simulink model "BierPong_02"  (R2021a)
settings: Solver=VariableStepAuto  StartTime=0.0  StopTime=5.0  RelTol=1e-3
model workspace (MAT data in the model file):
  c_w = 0.47
  d_Ball = 0.04
  d_cup = 0.095
  g = 9.81
  len = 2.1
  m_Ball = 2.7
  roh = 1.2
  s_cup = 0.05
settings Model: OrderedModelArguments=off  Creator=Max  LastModifiedBy=Max

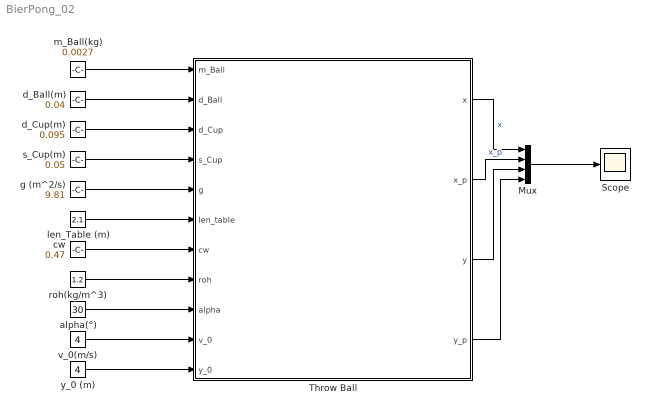
== system BierPong_02 ==
  Mux : Mux
  Scope : Scope
  Throw Ball : Subsystem
  alpha(°) : Constant  Value=30
  cw : Constant  Value=0.47
  d_Ball(m) : Constant  Value=0.04
  d_Cup(m) : Constant  Value=0.095
  g (m^2/s) : Constant  Value=9.81
  len_Table (m) : Constant  Value=2.1
  m_Ball(kg) : Constant  Value=0.0027
  roh(kg/m^3) : Constant  Value=1.2
  s_Cup(m) : Constant  Value=0.05
  v_0(m/s) : Constant  Value=4
  y_0 (m) : Constant  Value=4
  wires:
  m_Ball(kg)/1 -> Throw Ball/1(m_Ball)
  d_Ball(m)/1 -> Throw Ball/2(d_Ball)
  d_Cup(m)/1 -> Throw Ball/3(d_Cup)
  s_Cup(m)/1 -> Throw Ball/4(s_Cup)
  roh(kg/m^3)/1 -> Throw Ball/8(roh)
  cw/1 -> Throw Ball/7(cw)
  len_Table (m)/1 -> Throw Ball/6(len_table)
  g (m^2/s)/1 -> Throw Ball/5(g)
  Throw Ball/1(x) -> Mux/1  "x"
  Throw Ball/2(x_p) -> Mux/2  "x_p"
  Throw Ball/3(y) -> Mux/3
  Throw Ball/4(y_p) -> Mux/4
  Mux/1 -> Scope/1
  alpha(°)/1 -> Throw Ball/9(alpha)
  v_0(m/s)/1 -> Throw Ball/10(v_0)
  y_0 (m)/1 -> Throw Ball/11(y_0)

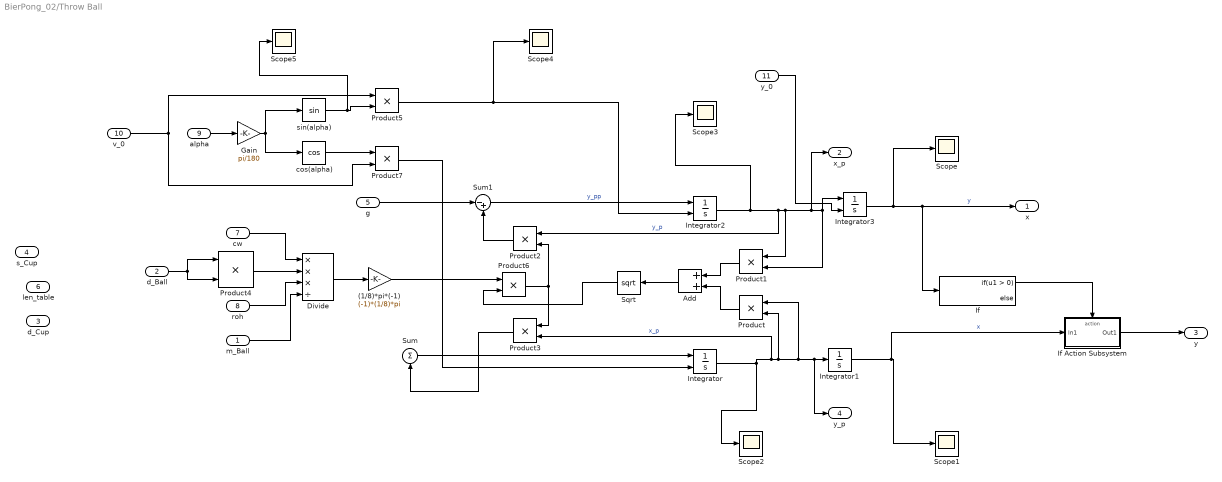
== system BierPong_02/Throw Ball ==
  m_Ball : Inport
  d_Ball : Inport  Port=2
  d_Cup : Inport  Port=3
  s_Cup : Inport  Port=4
  g : Inport  Port=5
  len_table : Inport  Port=6
  cw : Inport  Port=7
  roh : Inport  Port=8
  alpha : Inport  Port=9
  v_0 : Inport  Port=10
  y_0 : Inport  Port=11
  " sin(alpha)" : Trigonometry  OutputSignalType=real
  (1/8)*pi*(-1) : Gain  Gain=(-1)*(1/8)*pi
  Add : Sum
  Divide : Product  Inputs=***/
  Gain : Gain  Gain=pi/180
  If : If
  If Action Subsystem : Subsystem  TreatAsAtomicUnit=on
  Integrator : Integrator  InitialConditionSource=external  InitialCondition=2
  Integrator1 : Integrator  LimitOutput=on  LowerSaturationLimit=0
  Integrator2 : Integrator  InitialConditionSource=external  LimitOutput=on
  Integrator3 : Integrator  InitialConditionSource=external  InitialCondition=1  LimitOutput=on  LowerSaturationLimit=0
  Product{,1..7} (8 alike) : Product
  Scope{,1..5} (6 alike) : Scope
  Sqrt : Sqrt  SaturateOnIntegerOverflow=on
  Sum : Sum  Inputs=|+
  Sum1 : Sum  Inputs=|-+
  cos(alpha) : Trigonometry  Operator=cos
  x : Outport
  x_p : Outport  Port=2
  y : Outport  Port=3
  y_p : Outport  Port=4
  wires:
  Sum1/1 -> Integrator2/1  "y_pp"
  Product/1 -> Add/2
  Integrator2/1 -> Scope3/1, x_p/1, Integrator3/1, Product1/2, Product1/1, Product2/1  "y_p"
  Product2/1 -> Sum1/2
  Integrator/1 -> Product3/2, Product/2, Product/1, y_p/1, Integrator1/1, Scope2/1  "x_p"
  Product3/1 -> Sum/1
  Sqrt/1 -> Product6/2
  Product1/1 -> Add/1
  Add/1 -> Sqrt/1
  Product6/1 -> Product2/2, Product3/1
  d_Ball/1 -> Product4/2, Product4/1
  cw/1 -> Divide/1
  Divide/1 -> (1/8)*pi*(-1)/1
  (1/8)*pi*(-1)/1 -> Product6/1
  g/1 -> Sum1/1
  Sum/1 -> Integrator/1
  Product4/1 -> Divide/2
  roh/1 -> Divide/3
  m_Ball/1 -> Divide/4
  Integrator1/1 -> If Action Subsystem/1(In1), Scope1/1  "x"
  Integrator3/1 -> If/1, x/1, Scope/1  "y"
  If/1 -> If Action Subsystem/Action
  If Action Subsystem/1(Out1) -> y/1
  Gain/1 -> cos(alpha)/1, " sin(alpha)"/1
  v_0/1 -> Product7/2, Product5/1
  " sin(alpha)"/1 -> Scope5/1, Product5/2
  cos(alpha)/1 -> Product7/1
  Product5/1 -> Scope4/1, Integrator2/2
  Product7/1 -> Integrator/2
  y_0/1 -> Integrator3/2
  alpha/1 -> Gain/1

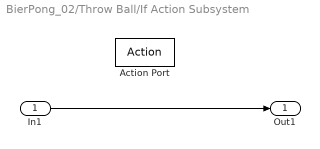
== system BierPong_02/Throw Ball/If Action Subsystem ==
  In1 : Inport
  Action Port : ActionPort  ActionPortLabel=if(u1 > 0)
  Out1 : Outport
  wires:
  In1/1 -> Out1/1
